simulink model "lqgsim"  (R2019b)
settings: Solver=VariableStepAuto  StartTime=0.0  StopTime=10.0  RelTol=1e-3
values from neighbouring files (symbols this model uses):
  C = eye(6)    [lqrController.m]    (also in luenberger_X.m; luenberger_X_t1_t2.m; luenberger_non_linear.m; simINIT.m = [1 0 0 0 0 0; 0 0 0 0 0 0; 0 0 0 0 0 0; 0 0 0 0 0 0; 0 0 0 0)
  Kr = lqr(A,B,Q,R)    [luenberger_non_linear.m]
  sysKF = ss(A-Kf*C,[B Kf],eye(6),0*[B Kf])    [simINIT.m]
settings Model: Creator=aadi0  LastModifiedBy=aadi0

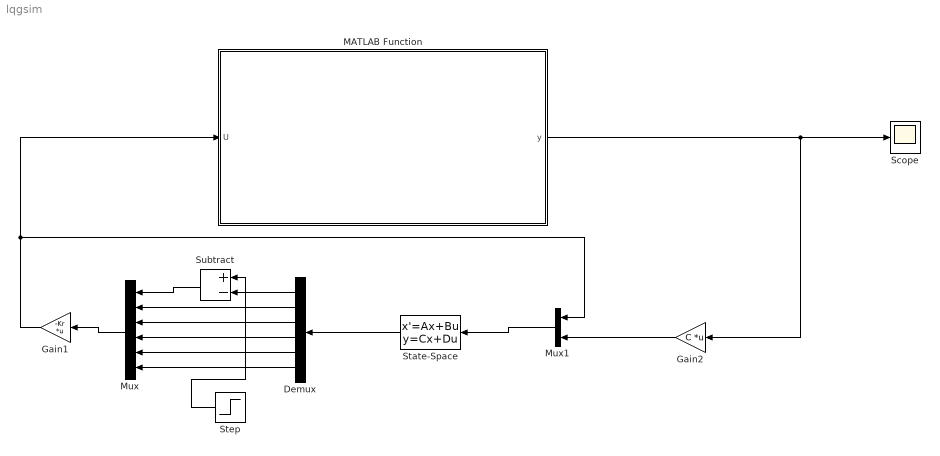
== system lqgsim ==
  Demux : Demux  Outputs=6
  Gain1 : Gain  Gain=-Kr  Multiplication=Matrix(K*u) (u vector)
  Gain2 : Gain  Gain=C  Multiplication=Matrix(K*u) (u vector)
  MATLAB Function : MATLAB Function  TreatAsAtomicUnit=on
  Mux : Mux  Inputs=6
  Mux1 : Mux  Inputs=2
  Scope : Scope
  State-Space : StateSpace  A=sysKF.A  B=sysKF.B  C=sysKF.C  D=sysKF.D  InitialCondition=[0 0 0 0 0 0]
  Step : Step  Time=2  After=2  SampleTime=0
  Subtract : Sum  Inputs=+-
  wires:
  Gain1/1 -> Mux1/1, MATLAB Function/1(U)
  Step/1 -> Subtract/1
  Subtract/1 -> Mux/1
  Demux/2 -> Mux/2
  Demux/3 -> Mux/3
  Demux/4 -> Mux/4
  Demux/5 -> Mux/5
  Demux/6 -> Mux/6
  Mux/1 -> Gain1/1
  Demux/1 -> Subtract/2
  MATLAB Function/1(y) -> Gain2/1, Scope/1
  Gain2/1 -> Mux1/2
  Mux1/1 -> State-Space/1
  State-Space/1 -> Demux/1

== matlab function lqgsim/MATLAB Function ==
  data: U input; y output size=[1 6]
function y  = nonlinear(U)
tspan = (0:1:100);
y = ones(1,6);
x0 = [-2;0;1;0;1;0];
[t,x]=ode45(@(t,x)nonlinearsolver(x,U),tspan,x0);
y(1) = x(1);
y(2) = x(2);
y(3) = x(3);
y(4) = x(4);
y(5) = x(5);
y(6) = x(6);
plot(t,x)
end

function dx = nonlinearsolver(x,U)
M = 1000;
m1 = 100;
m2 = 100;
l1 = 20;
l2 = 10;
g = 9.81;
dx = zeros(6,1);
x_ = (U(1) - m1*g*sin(x(3))*cos(x(3))-m2*g*sin(x(5))*cos(x(5))-l1*m1*(x(4)^2)*sin(x(3))-l2*m2*(x(6)^2)*sin(x(5)))/(M+m1*(sin(x(3))^2)+m2*sin(x(5)^2));
dx(1,1)= x(2);
dx(2,1)= x_;
dx(3,1)=x(4);
dx(4,1)= (x_*cos(x(3))-g*sin(x(3)))/l1;
dx(5,1)=x(6);
dx(6,1)= (x_*cos(x(5))-g*sin(x(5)))/l2;
end
